simulink model "InteriorLightController"  (R2021b)
settings: Solver=VariableStepAuto  StartTime=0.0  StopTime=10.0  RelTol=1e-3
settings Model: Creator=AGM4GA  LastModifiedBy=AGM4GA

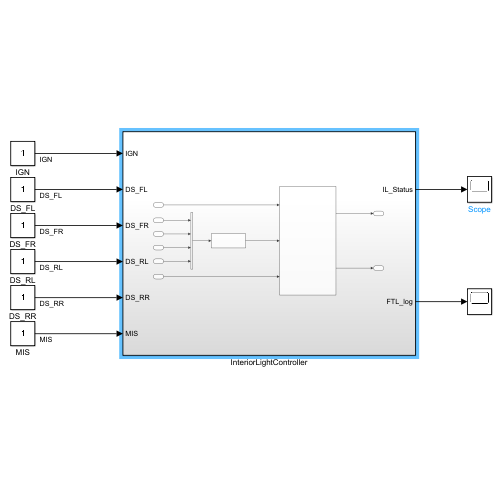
[thumbnail: Simulink's stored preview of the top-level diagram]
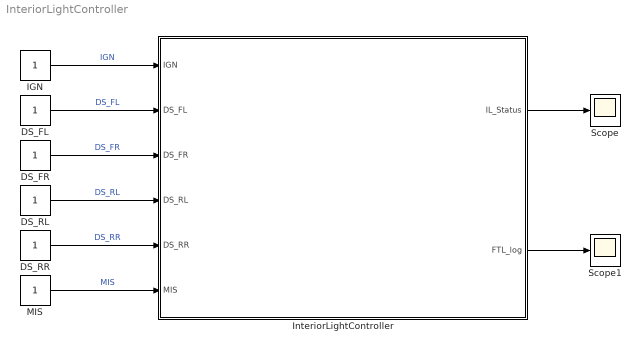
== system InteriorLightController ==
  DS_FL : Constant
  DS_FR : Constant
  DS_RL : Constant
  DS_RR : Constant
  IGN : Constant
  InteriorLightController : Subsystem
  MIS : Constant
  Scope : Scope
  Scope1 : Scope
  wires:
  IGN/1 -> InteriorLightController/1(IGN)  "IGN"
  DS_FL/1 -> InteriorLightController/2(DS_FL)  "DS_FL"
  DS_FR/1 -> InteriorLightController/3(DS_FR)  "DS_FR"
  DS_RL/1 -> InteriorLightController/4(DS_RL)  "DS_RL"
  DS_RR/1 -> InteriorLightController/5(DS_RR)  "DS_RR"
  MIS/1 -> InteriorLightController/6(MIS)  "MIS"
  InteriorLightController/1(IL_Status) -> Scope/1
  InteriorLightController/2(FTL_log) -> Scope1/1

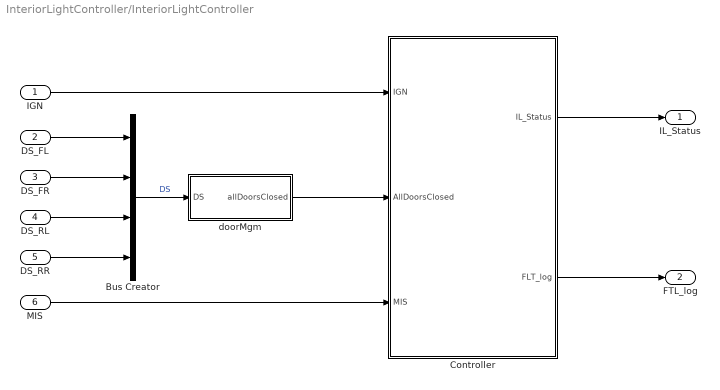
== system InteriorLightController/InteriorLightController ==
  IGN : Inport
  DS_FL : Inport  Port=2
  DS_FR : Inport  Port=3
  DS_RL : Inport  Port=4
  DS_RR : Inport  Port=5
  MIS : Inport  Port=6
  Bus Creator : BusCreator  Inputs=4
  Controller : Subsystem
  doorMgm : Subsystem
  IL_Status : Outport
  FTL_log : Outport  Port=2
  wires:
  Controller/2(FLT_log) -> FTL_log/1
  DS_RR/1 -> Bus Creator/4
  DS_FL/1 -> Bus Creator/1
  MIS/1 -> Controller/3(MIS)
  Controller/1(IL_Status) -> IL_Status/1
  DS_RL/1 -> Bus Creator/3
  doorMgm/1(allDoorsClosed) -> Controller/2(AllDoorsClosed)
  DS_FR/1 -> Bus Creator/2
  Bus Creator/1 -> doorMgm/1(DS)  "DS"
  IGN/1 -> Controller/1(IGN)

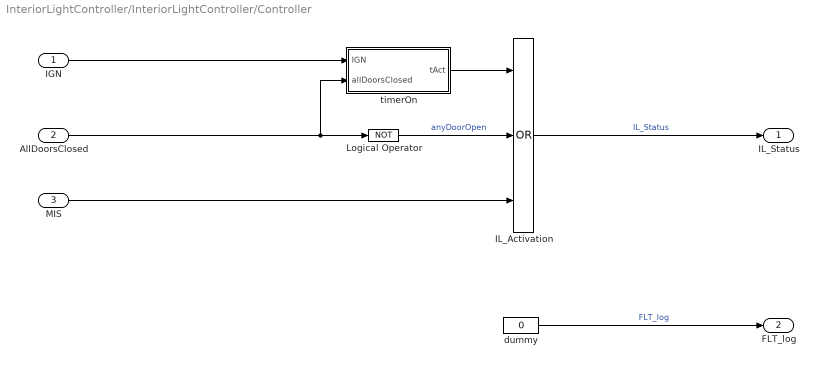
== system InteriorLightController/InteriorLightController/Controller ==
  IGN : Inport
  AllDoorsClosed : Inport  Port=2
  MIS : Inport  Port=3
  IL_Activation : Logic  Operator=OR  Inputs=3  AllPortsSameDT=off  OutDataTypeStr=boolean
  Logical Operator : Logic  Operator=NOT  AllPortsSameDT=off  OutDataTypeStr=boolean
  dummy : Constant  Value=0
  timerOn : Subsystem
  IL_Status : Outport
  FLT_log : Outport  Port=2
  wires:
  MIS/1 -> IL_Activation/3
  IL_Activation/1 -> IL_Status/1  "IL_Status"
  Logical Operator/1 -> IL_Activation/2  "anyDoorOpen"
  timerOn/1(tAct) -> IL_Activation/1
  AllDoorsClosed/1 -> timerOn/2(allDoorsClosed), Logical Operator/1
  IGN/1 -> timerOn/1(IGN)
  dummy/1 -> FLT_log/1  "FLT_log"

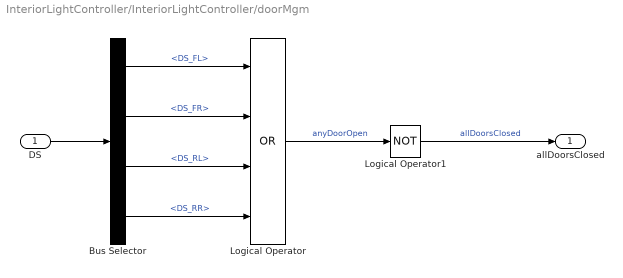
== system InteriorLightController/InteriorLightController/doorMgm ==
  DS : Inport
  Bus Selector : BusSelector  OutputSignals=DS_FL,DS_FR,DS_RL,DS_RR
  Logical Operator : Logic  Operator=OR  Inputs=4  AllPortsSameDT=off  OutDataTypeStr=boolean
  Logical Operator1 : Logic  Operator=NOT  AllPortsSameDT=off  OutDataTypeStr=boolean
  allDoorsClosed : Outport
  wires:
  DS/1 -> Bus Selector/1
  Bus Selector/4 -> Logical Operator/4  "<DS_RR>"
  Bus Selector/3 -> Logical Operator/3  "<DS_RL>"
  Bus Selector/2 -> Logical Operator/2  "<DS_FR>"
  Bus Selector/1 -> Logical Operator/1  "<DS_FL>"
  Logical Operator/1 -> Logical Operator1/1  "anyDoorOpen"
  Logical Operator1/1 -> allDoorsClosed/1  "allDoorsClosed"

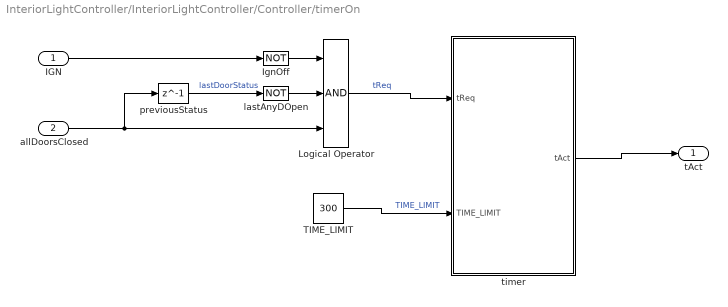
== system InteriorLightController/InteriorLightController/Controller/timerOn ==
  IGN : Inport
  allDoorsClosed : Inport  Port=2
  IgnOff : Logic  Operator=NOT  AllPortsSameDT=off  OutDataTypeStr=boolean
  Logical Operator : Logic  Inputs=3  AllPortsSameDT=off  OutDataTypeStr=boolean
  TIME_LIMIT : Constant  Value=300
  lastAnyDOpen : Logic  Operator=NOT  AllPortsSameDT=off  OutDataTypeStr=boolean
  previousStatus : Delay  DelayLength=1  InputProcessing=Columns as channels (frame based)
  timer : Stateflow chart  TreatAsAtomicUnit=on
  tAct : Outport
  wires:
  allDoorsClosed/1 -> Logical Operator/3, previousStatus/1
  previousStatus/1 -> lastAnyDOpen/1  "lastDoorStatus"
  lastAnyDOpen/1 -> Logical Operator/2
  Logical Operator/1 -> timer/1(tReq)  "tReq"
  timer/1(tAct) -> tAct/1
  IgnOff/1 -> Logical Operator/1
  IGN/1 -> IgnOff/1
  TIME_LIMIT/1 -> timer/2(TIME_LIMIT)  "TIME_LIMIT"

== stateflow chart InteriorLightController/Controller/timerOn/timer ==
  (default) -> (junction 40) : {t=0;}
  (junction 40) -> (junction 27) [order 1] : [tReq ==1 &&...
      | t < TIME_LIMIT]
  (junction 40) -> (junction 29) [order 2] : {t = 0;
      | tAct = 0;}
  (junction 27) -> (junction 36) : {t = t + 1;
      | tAct = 1;}
  (junction 36) -> (junction 29)
  (junction 29) -> (junction 33)
  data: tReq input; tAct output; TIME_LIMIT input; t local double size=1
